simulink model "TwoLinkPlanarRobotHybridControl_gen1"  (Simulink 7.9)
settings: Solver=ode1  StartTime=0.0  StopTime=10.0  FixedStep=0.01  RelTol=1e-3
values from neighbouring files (symbols this model uses):
  m = [1 1]    [FurutaPendulum_Dynamics.m]    (also in Question_2.m = [m_1 m_2]; test_ForwardDynamics.m = [1 1 1]; test_TwoLinkPlanarRobotDynamics.m = [m1 m2]; test_TwoLinkPlanarRobotHybridControl.m = [m1 m2])
  N = 5    [createEllipsoid.m]
  s = tf('s')    [Current_loop_bode.m]    (also in Question_1.m = 15)
undefined symbols (not defined in the file or in its folder): rad
libraries: mblibv1 x20, simulink x1
settings Model: Creator=leavesdown_admin  LastModifiedBy=leavesdown_admin
settings SimMechanicsCC: VisDuringSimulation=on
settings ConfigurationSet: Description=SimMechanics 2G

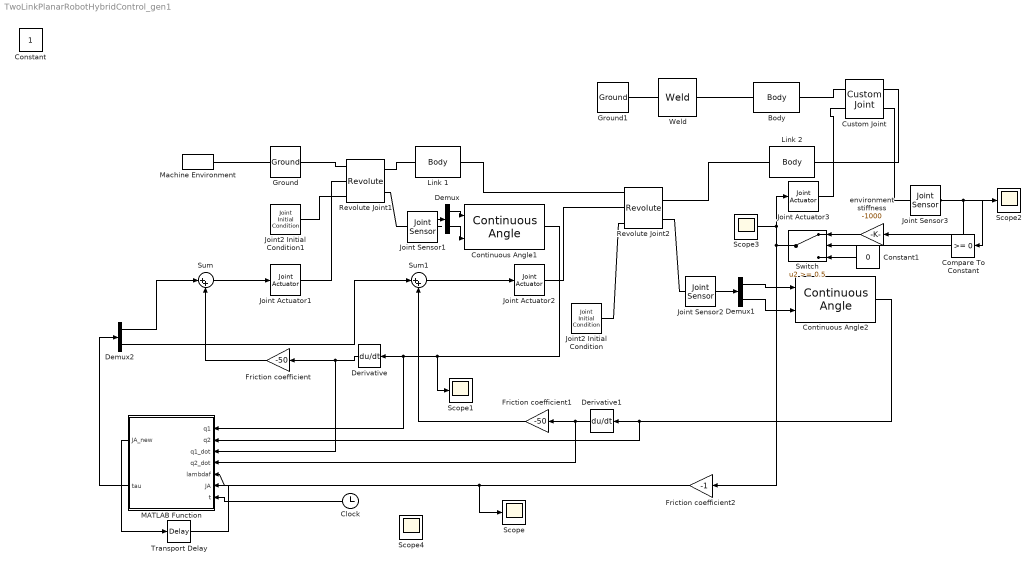
== system TwoLinkPlanarRobotHybridControl_gen1 ==
  Body : mblibv1/Bodies/Body  LConnTagsString=CS1  RConnTagsString=CS2  UpdateFromCAD=off  DialogClass=MechanicalBodyBlock  Mass=1  MassUnits=kg  InertiaUnits=kg*m^2  Inertia=eye(3)  Shape=Cylinder  ShapeDims=[1 1]  ShapeUnits=m  ShapeUse=false  Density=1  DensityUnits=kg/m^3  DensityUse=false  GraphicsMode=MACHINE_DEFAULT  BodyColorSelMode=MACHINE_DEFAULT  BodyColor=[1 0 0]  AttachedToCS=CG  CG=Left$CG$[1 1 0]$World$World$m$[0 0 0]$Euler X-Y-Z$deg$WORLD$false$none  WorkingFrames=Left$CS1$[0 2 0]$World$World$m$[0 0 0]$Euler X-Y-Z$deg$WORLD$true$none#Right$CS2$[2 0 0]$World$World$m$[0 0 0]$Euler X-Y-Z$deg$WORLD$true$none  CGPos=[1 1 0]  CGRot=[0 0 0]  CS0Pos=[]  CS0Rot=[]  CS1Pos=[0 2 0]  CS1Rot=[0 0 0]  CS2Pos=[2 0 0]  CS2Rot=[0 0 0]  CS3Pos=[]  CS3Rot=[]  CS4Pos=[]  CS4Rot=[]  CS5Pos=[]  CS5Rot=[]  CS6Pos=[]  CS6Rot=[]  CS7Pos=[]  CS7Rot=[]  CS8Pos=[]  CS8Rot=[]  CS9Pos=[]  CS9Rot=[]  CS10Pos=[]  CS10Rot=[]  CS11Pos=[]  CS11Rot=[]  CS12Pos=[]  CS12Rot=[]  CS13Pos=[]  CS13Rot=[]  CS14Pos=[]  CS14Rot=[]  CS15Pos=[]  CS15Rot=[]  CS16Pos=[]  CS16Rot=[]  CS17Pos=[]  CS17Rot=[]  CS18Pos=[]  CS18Rot=[]  CS19Pos=[]  CS19Rot=[]  CS20Pos=[]  CS20Rot=[]
  Clock : Clock
  Compare To Constant : simulink/Logic and Bit Operations/Compare To Constant  relop=>=  const=0  OutDataTypeStr=uint8
  Constant1 : Constant  Value=0
  Continuous Angle1 : mblibv1/Utilities/Continuous Angle  rad=rad  rads=rad/s
  Continuous Angle2 : mblibv1/Utilities/Continuous Angle  rad=rad  rads=rad/s
  Custom Joint : mblibv1/Joints/Custom Joint  LConnTagsString=__newl0|SA1  RConnTagsString=__newr0|SA1  UpdateFromCAD=off  NumSAPorts=2  CutJoint=off  MarkAsCut=off  Primitives=prismatic  PrimitiveProps=P1$World$[sqrt(2)/2 sqrt(2)/2 0]$Prismatic#P3$World$[-sqrt(2)/2 sqrt(2)/2 0]$Prismatic#R1$World$[1 0 0]$Revolute#R2$World$[0 1 0]$Revolute#R3$World$[0 0 1]$Revolute#P2$World$[0 0 1]$Prismatic  DialogClass=JointBlock  R1Axis=[1 0 0]  R2Axis=[0 1 0]  R3Axis=[0 0 1]  P1Axis=[sqrt(2)/2 sqrt(2)/2 0]  P2Axis=[0 0 1]  P3Axis=[-sqrt(2)/2 sqrt(2)/2 0]  SAxis=[]
  Demux : Demux  Outputs=2
  Demux1 : Demux  Outputs=2
  Demux2 : Demux  Outputs=2
  Derivative : Derivative
  Derivative1 : Derivative
  Friction coefficient : Gain  Gain=-50
  Friction coefficient1 : Gain  Gain=-50
  Friction coefficient2 : Gain  Gain=-1
  Ground : mblibv1/Bodies/Ground  UpdateFromCAD=off  LeftPortType=env  RightPortType=workingframe  PhysicalDomain=Mechanical  DialogClass=GroundBlock  CoordPosition=[0 0 0]  CoordPositionUnits=m  StateVectorMgrId=-1  MachineId=[0 0]  ShowEnvPort=on
  Ground1 : mblibv1/Bodies/Ground  UpdateFromCAD=off  LeftPortType=env  RightPortType=workingframe  PhysicalDomain=Mechanical  DialogClass=GroundBlock  CoordPosition=[0 2 0]  CoordPositionUnits=m  StateVectorMgrId=-1  MachineId=[0 0]  ShowEnvPort=off
  Joint Actuator1 : mblibv1/Sensors &  Actuators/Joint Actuator  UpdateFromCAD=off  PhysicalDomain=Mechanical  PortType=blob  ActuationStyle=Force  AngleUnits=deg  ArcVelocityUnits=deg/s  ArcAccelerationUnits=deg/s^2  CoordPositionUnits=m  VelocityUnits=m/s  AccelerationUnits=m/s^2  ForceUnits=N  TorqueUnits=N*m  ActiveIO=on  Width=1  DialogClass=MechanicalActuatorBlock  Primitive=R1  ReferenceFrame=Absolute (World)
  Joint Actuator2 : mblibv1/Sensors &  Actuators/Joint Actuator  UpdateFromCAD=off  PhysicalDomain=Mechanical  PortType=blob  ActuationStyle=Force  AngleUnits=deg  ArcVelocityUnits=deg/s  ArcAccelerationUnits=deg/s^2  CoordPositionUnits=m  VelocityUnits=m/s  AccelerationUnits=m/s^2  ForceUnits=N  TorqueUnits=N*m  ActiveIO=on  Width=1  DialogClass=MechanicalActuatorBlock  Primitive=R1  ReferenceFrame=Absolute (World)
  Joint Actuator3 : mblibv1/Sensors &  Actuators/Joint Actuator  UpdateFromCAD=off  PhysicalDomain=Mechanical  PortType=blob  ActuationStyle=Force  AngleUnits=deg  ArcVelocityUnits=deg/s  ArcAccelerationUnits=deg/s^2  CoordPositionUnits=m  VelocityUnits=m/s  AccelerationUnits=m/s^2  ForceUnits=N  TorqueUnits=N*m  ActiveIO=on  Width=1  DialogClass=MechanicalActuatorBlock  Primitive=P1  ReferenceFrame=Absolute (World)
  Joint Sensor1 : mblibv1/Sensors &  Actuators/Joint Sensor  UpdateFromCAD=off  PhysicalDomain=Mechanical  PortType=blob  Muxed=on  Pose=off  Angle=on  AngleUnits=rad  ArcVelocity=on  ArcVelocityUnits=rad/s  ArcAcceleration=off  ArcAccelerationUnits=deg/s^2  CoordPosition=on  CoordPositionUnits=m  Velocity=off  VelocityUnits=m/s  Acceleration=off  AccelerationUnits=m/s^2  Quaternion=on  QuaternionDT=off  QuaternionDDT=off  QuaternionUnits=off  OutputVector=[1]  ActiveIO=on  Width=2  DialogClass=MechanicalSensorBlock  Primitive=R1  Force=off  ForceUnits=N  Torque=off  TorqueUnits=N*m  ReferenceFrame=Absolute (World)  ReactionSensedSide=Base  ReactionReferenceFrame=Absolute (World)  ReactionForce=off  ReactionForceUnits=N  ReactionMoment=off  ReactionMomentUnits=N*m
  Joint Sensor2 : mblibv1/Sensors &  Actuators/Joint Sensor  UpdateFromCAD=off  PhysicalDomain=Mechanical  PortType=blob  Muxed=on  Pose=off  Angle=on  AngleUnits=rad  ArcVelocity=on  ArcVelocityUnits=rad/s  ArcAcceleration=off  ArcAccelerationUnits=deg/s^2  CoordPosition=on  CoordPositionUnits=m  Velocity=off  VelocityUnits=m/s  Acceleration=off  AccelerationUnits=m/s^2  Quaternion=on  QuaternionDT=off  QuaternionDDT=off  QuaternionUnits=off  OutputVector=[1]  ActiveIO=on  Width=2  DialogClass=MechanicalSensorBlock  Primitive=R1  Force=off  ForceUnits=N  Torque=off  TorqueUnits=N*m  ReferenceFrame=Absolute (World)  ReactionSensedSide=Base  ReactionReferenceFrame=Absolute (World)  ReactionForce=off  ReactionForceUnits=N  ReactionMoment=off  ReactionMomentUnits=N*m
  Joint Sensor3 : mblibv1/Sensors &  Actuators/Joint Sensor  UpdateFromCAD=off  PhysicalDomain=Mechanical  PortType=blob  Muxed=on  Pose=off  Angle=on  AngleUnits=rad  ArcVelocity=on  ArcVelocityUnits=rad/s  ArcAcceleration=off  ArcAccelerationUnits=deg/s^2  CoordPosition=on  CoordPositionUnits=m  Velocity=off  VelocityUnits=m/s  Acceleration=off  AccelerationUnits=m/s^2  Quaternion=on  QuaternionDT=off  QuaternionDDT=off  QuaternionUnits=off  OutputVector=[1]  ActiveIO=on  Width=1  DialogClass=MechanicalSensorBlock  Primitive=P1  Force=off  ForceUnits=N  Torque=off  TorqueUnits=N*m  ReferenceFrame=Absolute (World)  ReactionSensedSide=Base  ReactionReferenceFrame=Absolute (World)  ReactionForce=off  ReactionForceUnits=N  ReactionMoment=off  ReactionMomentUnits=N*m
  Joint2 Initial Condition : mblibv1/Sensors &  Actuators/Joint Initial Condition  UpdateFromCAD=off  LeftPortType=blob  RightPortType=blob  PhysicalDomain=mechanical  DialogClass=InitialConditionBlock  InitialConditions=P1$false$0$m$deg$0$m/s$deg/s#P2$false$0$m$deg$0$m/s$deg/s#P3$false$0$m$deg$0$m/s$deg/s#R1$true$pi/2$m$rad$0$m/s$rad/s#R2$false$0$m$deg$0$m/s$deg/s#R3$false$0$m$deg$0$m/s$deg/s#S$false$0$m$deg$0$m/s$deg/s  P1PIC=0  P1VIC=0  P2PIC=0  P2VIC=0  P3PIC=0  P3VIC=0  R1PIC=pi/2  R1VIC=0  R2PIC=0  R2VIC=0  R3PIC=0  R3VIC=0  SPIC=0  SVIC=0
  Joint2 Initial Condition1 : mblibv1/Sensors &  Actuators/Joint Initial Condition  UpdateFromCAD=off  LeftPortType=blob  RightPortType=blob  PhysicalDomain=mechanical  DialogClass=InitialConditionBlock  InitialConditions=P1$false$0$m$deg$0$m/s$deg/s#P2$false$0$m$deg$0$m/s$deg/s#P3$false$0$m$deg$0$m/s$deg/s#R1$true$0$m$rad$0$m/s$rad/s#R2$false$0$m$deg$0$m/s$deg/s#R3$false$0$m$deg$0$m/s$deg/s#S$false$0$m$deg$0$m/s$deg/s  P1PIC=0  P1VIC=0  P2PIC=0  P2VIC=0  P3PIC=0  P3VIC=0  R1PIC=0  R1VIC=0  R2PIC=0  R2VIC=0  R3PIC=0  R3VIC=0  SPIC=0  SVIC=0
  Link 1 : mblibv1/Bodies/Body  LConnTagsString=CS1  RConnTagsString=CS2  UpdateFromCAD=off  DialogClass=MechanicalBodyBlock  Mass=50  MassUnits=kg  InertiaUnits=kg*m^2  Inertia=[0 0 0;0 10 0;0 0 10];  Shape=Cylinder  ShapeDims=[1 1]  ShapeUnits=m  ShapeUse=false  Density=1  DensityUnits=kg/m^3  DensityUse=false  GraphicsMode=MACHINE_DEFAULT  BodyColorSelMode=COLORPALETTE  BodyColor=[1 0 0]  AttachedToCS=CG  CG=Left$CG$[-0.5 0 0]$CS2$CS2$m$eye(3)$3x3 Transform$rad$CS2$false$none  WorkingFrames=Left$CS1$[0 0 0]$Adjoining$Adjoining$m$eye(3)$3x3 Transform$rad$Adjoining$true$none#Right$CS2$[1 0 0]$CS1$CS1$m$eye(3)$3x3 Transform$rad$CS1$true$none  CGPos=[-0.5 0 0]  CGRot=eye(3)  CS0Pos=[]  CS0Rot=[]  CS1Pos=[0 0 0]  CS1Rot=eye(3)  CS2Pos=[1 0 0]  CS2Rot=eye(3)  CS3Pos=[]  CS3Rot=[]  CS4Pos=[]  CS4Rot=[]  CS5Pos=[]  CS5Rot=[]  CS6Pos=[]  CS6Rot=[]  CS7Pos=[]  CS7Rot=[]  CS8Pos=[]  CS8Rot=[]  CS9Pos=[]  CS9Rot=[]  CS10Pos=[]  CS10Rot=[]  CS11Pos=[]  CS11Rot=[]  CS12Pos=[]  CS12Rot=[]  CS13Pos=[]  CS13Rot=[]  CS14Pos=[]  CS14Rot=[]  CS15Pos=[]  CS15Rot=[]  CS16Pos=[]  CS16Rot=[]  CS17Pos=[]  CS17Rot=[]  CS18Pos=[]  CS18Rot=[]  CS19Pos=[]  CS19Rot=[]  CS20Pos=[]  CS20Rot=[]
  Link 2 : mblibv1/Bodies/Body  LConnTagsString=CS1  RConnTagsString=CS2  UpdateFromCAD=off  DialogClass=MechanicalBodyBlock  Mass=50  MassUnits=kg  InertiaUnits=kg*m^2  Inertia=[0 0 0;0 10 0;0 0 10];  Shape=Cylinder  ShapeDims=[1 1]  ShapeUnits=m  ShapeUse=false  Density=1  DensityUnits=kg/m^3  DensityUse=false  GraphicsMode=MACHINE_DEFAULT  BodyColorSelMode=MACHINE_DEFAULT  BodyColor=[1 0 0]  AttachedToCS=CG  CG=Left$CG$[-0.5 0 0]$CS2$CS2$m$eye(3)$3x3 Transform$rad$CS2$false$none  WorkingFrames=Left$CS1$[0 0 0]$Adjoining$Adjoining$m$eye(3)$3x3 Transform$rad$Adjoining$true$none#Right$CS2$[1 0 0]$CS1$CS1$m$eye(3)$3x3 Transform$rad$CS1$true$none  CGPos=[-0.5 0 0]  CGRot=eye(3)  CS0Pos=[]  CS0Rot=[]  CS1Pos=[0 0 0]  CS1Rot=eye(3)  CS2Pos=[1 0 0]  CS2Rot=eye(3)  CS3Pos=[]  CS3Rot=[]  CS4Pos=[]  CS4Rot=[]  CS5Pos=[]  CS5Rot=[]  CS6Pos=[]  CS6Rot=[]  CS7Pos=[]  CS7Rot=[]  CS8Pos=[]  CS8Rot=[]  CS9Pos=[]  CS9Rot=[]  CS10Pos=[]  CS10Rot=[]  CS11Pos=[]  CS11Rot=[]  CS12Pos=[]  CS12Rot=[]  CS13Pos=[]  CS13Rot=[]  CS14Pos=[]  CS14Rot=[]  CS15Pos=[]  CS15Rot=[]  CS16Pos=[]  CS16Rot=[]  CS17Pos=[]  CS17Rot=[]  CS18Pos=[]  CS18Rot=[]  CS19Pos=[]  CS19Rot=[]  CS20Pos=[]  CS20Rot=[]
  MATLAB Function : MATLAB Function  TreatAsAtomicUnit=on
  Machine Environment : mblibv1/Bodies/Machine Environment  PortType=env  PhysicalDomain=Mechanical  DialogTemplateClass=MECH.MachineEnvironment  SyncWhenCopied=off  Gravity=[0 -9.81 0]  GravityUnits=m/s^2  GravityAsSignal=off  Dimensionality=Auto-detect  AnalysisType=Forward dynamics  LinearAssemblyTolerance=1e-3  LinearAssemblyToleranceUnits=m  AngularAssemblyTolerance=1e-3  AngularAssemblyToleranceUnits=rad  ConstraintSolverType=Stabilizing  ConstraintRelTolerance=1e-4  ConstraintAbsTolerance=1e-4  UseRobustSingularityHandling=off  RedundancyAnalysisToleranceType=Automatically select tolerance  RedundancyAnalysisTolerance=1e-14  StatePerturbationType=Fixed  PerturbationSize=1e-5  VisualizeMachine=on  BodyVisualizationType=Use model default body geometries  BodyColorSelMode=Use model default  DefaultBodyColor=[1 0 0]
  Revolute Joint1 : mblibv1/Joints/Revolute  LConnTagsString=__newl0|SA1|SA2  RConnTagsString=__newr0|SA1  UpdateFromCAD=off  NumSAPorts=3  CutJoint=off  MarkAsCut=off  Primitives=prismatic  PrimitiveProps=R1$Base$[0 0 1]$revolute  DialogClass=JointBlock  R1Axis=[0 0 1]
  Revolute Joint2 : mblibv1/Joints/Revolute  LConnTagsString=__newl0|SA1|SA2  RConnTagsString=__newr0|SA1  UpdateFromCAD=off  NumSAPorts=3  CutJoint=off  MarkAsCut=off  Primitives=prismatic  PrimitiveProps=R1$Base$[0 0 1]$revolute  DialogClass=JointBlock  R1Axis=[0 0 1]
  Scope{,1..4} (5 alike) : Scope
      Scope settings: YMin=14.5  YMax=23.5
      Scope1 settings: YMin=0.7  YMax=2.4
      Scope2 settings: YMin=-1.9  YMax=-1.15  SaveName=ScopeData2
      Scope3 settings: YMin=-1.9  YMax=-1.15  SaveName=ScopeData3
      Scope4 settings: YMin=-21  YMax=-19  SaveName=ScopeData4
  Sum : Sum  Inputs=|++
  Sum1 : Sum  Inputs=|++
  Switch : Switch  Threshold=0.5
  Transport Delay : TransportDelay  DelayTime=0.01
  Weld : mblibv1/Joints/Weld  LConnTagsString=__newl0  RConnTagsString=__newr0  UpdateFromCAD=off  NumSAPorts=0  CutJoint=off  MarkAsCut=off  Primitives=weld  PrimitiveProps=W$World$[0 0 0]$weld  DialogClass=JointBlock  WAxis=[0 0 0]
  environment stiffness : Gain  Gain=-1000
  Constant : Constant  IOType=siggen
  wires:
  Sum/1 -> Joint Actuator1/1
  Friction coefficient/1 -> Sum/2
  Sum1/1 -> Joint Actuator2/1
  Friction coefficient1/1 -> Sum1/2
  Derivative1/1 -> Friction coefficient1/1, MATLAB Function/4(q2_dot)
  Derivative/1 -> Friction coefficient/1, MATLAB Function/3(q1_dot)
  Joint Sensor1/1 -> Demux/1
  Demux/1 -> Continuous Angle1/1
  Demux/2 -> Continuous Angle1/2
  Continuous Angle1/1 -> Derivative/1, MATLAB Function/1(q1), Scope1/1
  Joint Sensor2/1 -> Demux1/1
  Demux1/1 -> Continuous Angle2/1
  Demux1/2 -> Continuous Angle2/2
  Continuous Angle2/1 -> Derivative1/1, MATLAB Function/2(q2)
  Clock/1 -> MATLAB Function/7(t)
  MATLAB Function/2(tau) -> Demux2/1
  Demux2/1 -> Sum/1
  Demux2/2 -> Sum1/1
  Joint Sensor3/1 -> Scope2/1, Compare To Constant/1, environment stiffness/1
  Compare To Constant/1 -> Switch/2
  environment stiffness/1 -> Switch/1
  Constant1/1 -> Switch/3
  Switch/1 -> Joint Actuator3/1, Scope3/1, Friction coefficient2/1
  Friction coefficient2/1 -> MATLAB Function/5(lambdaf), Scope/1
  MATLAB Function/1(JA_new) -> Transport Delay/1
  Transport Delay/1 -> MATLAB Function/6(JA)
  connections:
  Ground/RConn1 -- Revolute Joint1/LConn1
  Revolute Joint1/RConn1 -- Link 1/LConn1
  Machine Environment/RConn1 -- Ground/LConn1
  Revolute Joint2/LConn1 -- Link 1/RConn1
  Revolute Joint2/RConn1 -- Link 2/LConn1
  Joint Sensor1/LConn1 -- Revolute Joint1/RConn2
  Revolute Joint2/RConn2 -- Joint Sensor2/LConn1
  Joint Actuator1/RConn1 -- Revolute Joint1/LConn2
  Joint Actuator2/RConn1 -- Revolute Joint2/LConn2
  Joint2 Initial Condition/RConn1 -- Revolute Joint2/LConn3
  Joint2 Initial Condition1/RConn1 -- Revolute Joint1/LConn3
  Ground1/RConn1 -- Weld/LConn1
  Weld/RConn1 -- Body/LConn1
  Body/RConn1 -- Custom Joint/LConn1
  Joint Sensor3/LConn1 -- Custom Joint/RConn2
  Link 2/RConn1 -- Custom Joint/RConn1
  Joint Actuator3/RConn1 -- Custom Joint/LConn2

== matlab function MATLAB Function ==
  data: JA_new output double; q1 input double; q2 input double; q1_dot input double; q2_dot input double; lambdaf input double; JA input double; tau output double; t input double
function [JA_new,tau]  = fcn(q1,q2,q1_dot,q2_dot,lambdaf,JA,t)
coder.extrinsic('Newton_Euler_Iteration');
coder.extrinsic('Jacobian');
coder.extrinsic('Forward_Kinematics');

q=[q1;q2];
q_dot=[q1_dot;q2_dot];
Jtype=[0;0];
    a1=1;a2=1;
    n=2;%number of joints
    m1=50;m2=50;
    m=[m1 m2]; %define mass constants
    Il1=10;Il2=10;
    I=zeros(3,3,2);
    I(:,:,1)=[0 0 0;0 Il1 0;0 0 Il1];I(:,:,2)=[0 0 0;0 Il2 0;0 0 Il2];%define inertia tensor
    l1=0.5;l2=0.5;
    r_C=[[l1-a1;0;0] [l2-a2;0;0]];%define com coordinates of each link
    kv=[50;50];%define viscous friction constants
    g=9.8;
    g0=[0;-g;0];%define gravity vector
    lambdafd=20;%desired contact force
    DH=[[0;q1;a1;0] [0;q2;a2;0]];
    B=zeros(2,2);
    for i=1:n
        q_ddot_temp=[0;0];
        q_ddot_temp(i)=1;
        B(:,i) = Newton_Euler_Iteration(DH, m, I, r_C, Jtype, [0;0], q_ddot_temp, [0;0;0]);
    end
    Coriolis_Gravity=zeros(2,1);
    Coriolis_Gravity=Newton_Euler_Iteration(DH, m, I, r_C, Jtype, q_dot, [0;0], g0);%compute C(q,\dot{q})\dot{q}+G(q)
    
    J=zeros(6,n);
    J=Jacobian(DH,Jtype);
    Sf=[cos(pi/4);sin(pi/4)];
    Sv=[-sin(pi/4);cos(pi/4)];
    JA_new=J(1:2,:);
    dt=0.01;
    JA_dot=(JA_new-JA)./dt;
    Bm=50;Dm=400;Km=10;
    A_lump=zeros(4,4,n);
    A_lump = Forward_Kinematics(DH);
    Ae=A_lump(:,:,n);
    temp=[Sf Sv]'*[Ae(1,4);Ae(2,4)];
    sf=temp(1);sv=temp(2);    
    temp=[Sf Sv]'*JA*q_dot;
    sf_dot=temp(1);sv_dot=temp(2);
    sfc=sqrt(2);
    lambdav=0;% friction force in unconstrained direction is zero
    
    %desired trajectory in unconstrained direction
    svd=0.5*sin(2*pi/2*t);
    svd_dot=0.5*2*pi/2*cos(2*pi/2*t);
    svd_ddot=-0.5*(2*pi/2)^2*sin(2*pi/2*t);
    
    %position control law in unconstrained direction
    ev=sv-svd;
    ev_dot=sv_dot-svd_dot;
    Kp=25;Kd=5;
    av=svd_ddot-Kp*ev-Kd*ev_dot;
    
    %direct force control in constrained direction
    k_hat=1000;%estimation of contact stiffness k
    %calculate the estimate of velocity in the constrained direction
    %(lambdaf_dot)
    if sf<sfc
        lambdaf_dot_hat=0;
    else
        lambdaf_dot_hat=k_hat*sf_dot;
    end
    kp=25;kd=5;
    af=-kp/k_hat*(lambdaf-lambdafd)-kd/k_hat*lambdaf_dot_hat;
    
    % impedance control in constrained direction
%     Mm=50;Dm=400;Km=10;
%     sfd=sfc+lambdafd/Km;
%     af=1/Mm*(-Dm*(sf_dot)-Km*(sf-sfd)-lambdaf);
    
    %total control law
    tau=Coriolis_Gravity+kv.*q_dot+JA'*(Sf*lambdaf+Sv*lambdav)+B*JA'*inv(JA*JA'+0.01.*eye(2))*(-JA_dot*q_dot+Sf*af+Sv*av);
